simulink model "Umisteni_polu_integrator"  (R2024b)
settings: Solver=VariableStepAuto  StartTime=0.0  StopTime=10.0  RelTol=1e-3
values from neighbouring files (symbols this model uses):
  A = [0  1; -2  -3]    [Ackermann.m]    (also in Umisteni_polu_integrator.m = [0 1; -k/m -b/m])
  B = [0; 1]    [Ackermann.m]    (also in Umisteni_polu_integrator.m = [0; 1/m])
  C = [1 0]    [Umisteni_polu_integrator.m]
  K_i = K(3)    [Umisteni_polu_integrator.m]
  K_x = K(1:2)    [Umisteni_polu_integrator.m]
settings Model: Creator=mhusa  LastModifiedBy=mhusa

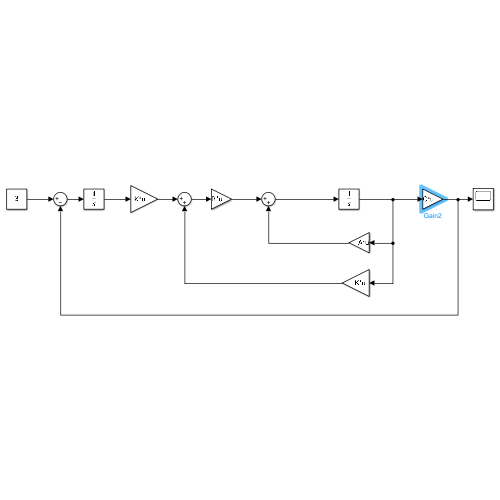
[thumbnail: Simulink's stored preview of the top-level diagram]
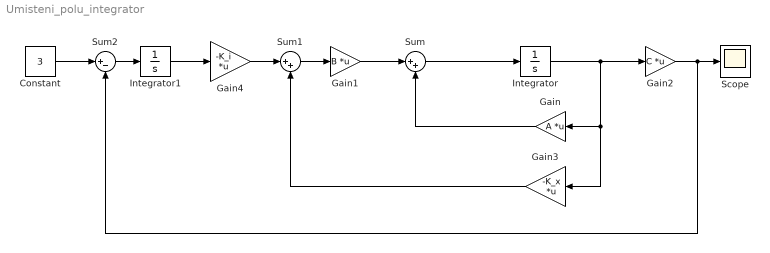
== system Umisteni_polu_integrator ==
  Constant : Constant  Value=3
  Gain : Gain  Gain=A  Multiplication=Matrix(K*u)
  Gain1 : Gain  Gain=B  Multiplication=Matrix(K*u)
  Gain2 : Gain  Gain=C  Multiplication=Matrix(K*u)
  Gain3 : Gain  Gain=-K_x  Multiplication=Matrix(K*u)
  Gain4 : Gain  Gain=-K_i  Multiplication=Matrix(K*u)
  Integrator : Integrator
  Integrator1 : Integrator
  Scope : Scope
  Sum : Sum  Inputs=|++
  Sum1 : Sum  Inputs=|++
  Sum2 : Sum  Inputs=|+-
  wires:
  Gain/1 -> Sum/2
  Sum/1 -> Integrator/1
  Gain1/1 -> Sum/1
  Integrator/1 -> Gain3/1, Gain/1, Gain2/1
  Gain3/1 -> Sum1/2
  Sum1/1 -> Gain1/1
  Gain4/1 -> Sum1/1
  Integrator1/1 -> Gain4/1
  Sum2/1 -> Integrator1/1
  Gain2/1 -> Sum2/2, Scope/1
  Constant/1 -> Sum2/1
